simulink model "task2"  (R2024a)
settings: Solver=VariableStepAuto  StartTime=0.0  StopTime=10  RelTol=1e-3
settings Model: Creator=lalayants  LastModifiedBy=lalayants

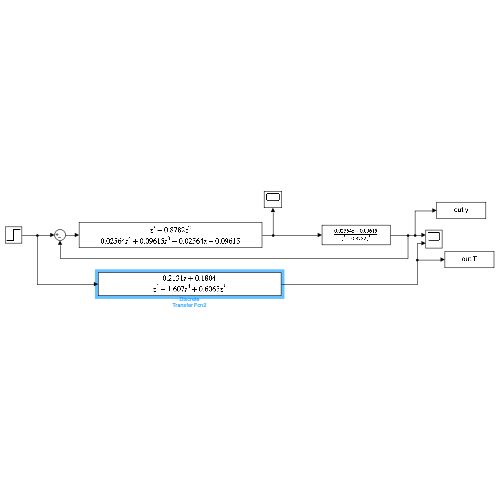
[thumbnail: Simulink's stored preview of the top-level diagram]
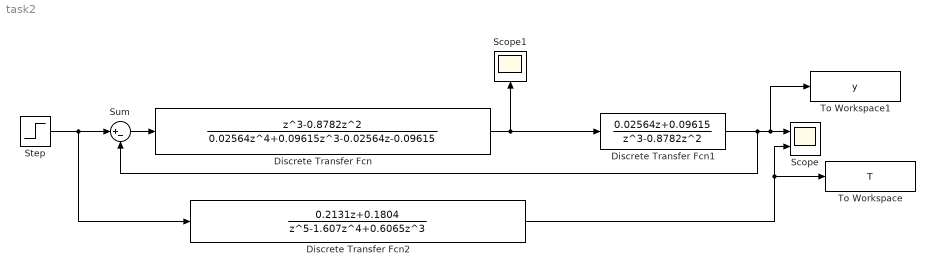
== system task2 ==
  Discrete Transfer Fcn : DiscreteTransferFcn  Numerator=[1 -0.8782 0 0]  Denominator=[0.02564 0.09615 0 -0.02564 -0.09615]
  Discrete Transfer Fcn1 : DiscreteTransferFcn  Numerator=[0.02564 0.09615]  Denominator=[1 -0.8782 0 0]
  Discrete Transfer Fcn2 : DiscreteTransferFcn  Numerator=[0.2131 0.1804]  Denominator=[1 -1.607 0.6065 0 0 0]
  Scope : Scope  NumInputPorts=2
  Scope1 : Scope
  Step : Step  Time=0  SampleTime=0
  Sum : Sum  Inputs=|+-
  To Workspace : ToWorkspace  VariableName=T  SaveFormat=Timeseries  SampleTime=-1
  To Workspace1 : ToWorkspace  VariableName=y  SaveFormat=Timeseries  SampleTime=-1
  wires:
  Step/1 -> Discrete Transfer Fcn2/1, Sum/1
  Discrete Transfer Fcn1/1 -> To Workspace1/1, Scope/1, Sum/2
  Sum/1 -> Discrete Transfer Fcn/1
  Discrete Transfer Fcn2/1 -> To Workspace/1, Scope/2
  Discrete Transfer Fcn/1 -> Discrete Transfer Fcn1/1, Scope1/1
